simulink model "SingleStreamSSRwithPL"  (R2024a)
settings: Solver=VariableStepAuto  StartTime=0.0  StopTime=pow2(12)  RelTol=1e-3
PreLoadFcn:
  | xmcCheckSlxPath(bdroot);
  | SSR4withPL_init;
InitFcn:
  | xmcCheckSlxPath(bdroot);
  | SSR4withPL_init;
values from neighbouring files (symbols this model uses):
  SHIFT_ACC = 15    [SSR4withPL_init.m]
  T = N    (= 8)    [SSR4withPL_init.m]
  Taps = NormalizeCoef(UTaps,32768)    [SSR4withPL_init.m]
  VectorSize = FramesPerVector*N    (= 32)    [SSR4withPL_init.m]
undefined symbols (not defined in the file or in its folder): c, FIR_MultiKernel_cin, FIR_MultiKernel_cincout, FIR_MultiKernel_cout, S, SingleStream, vsva2197, xcvc1902
libraries: aieBasic x40, hdlBasic x40, aieUtilities x32, hdlUtilities x24, dspobslib x1, simulink x1, vmcUtilities x1
(part 1 of 3)
settings Model: Creator=oliviert  LastModifiedBy=robg
settings SolverCC: AlgebraicLoopSolver=TrustRegion
settings DebuggingCC: AlgebraicLoopMsg=none  UnconnectedInputMsg=warning  UnconnectedOutputMsg=warning  UnconnectedLineMsg=warning
settings ModelReferenceCC: EnableRefExpFcnMdlSchedulingChecks=on
settings RTWCC: GPUComputeCapability=3.5  DLArmComputeVersion=19.05

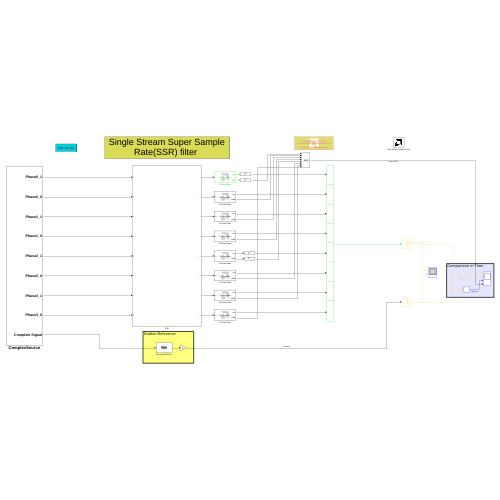
[thumbnail: Simulink's stored preview of the top-level diagram]
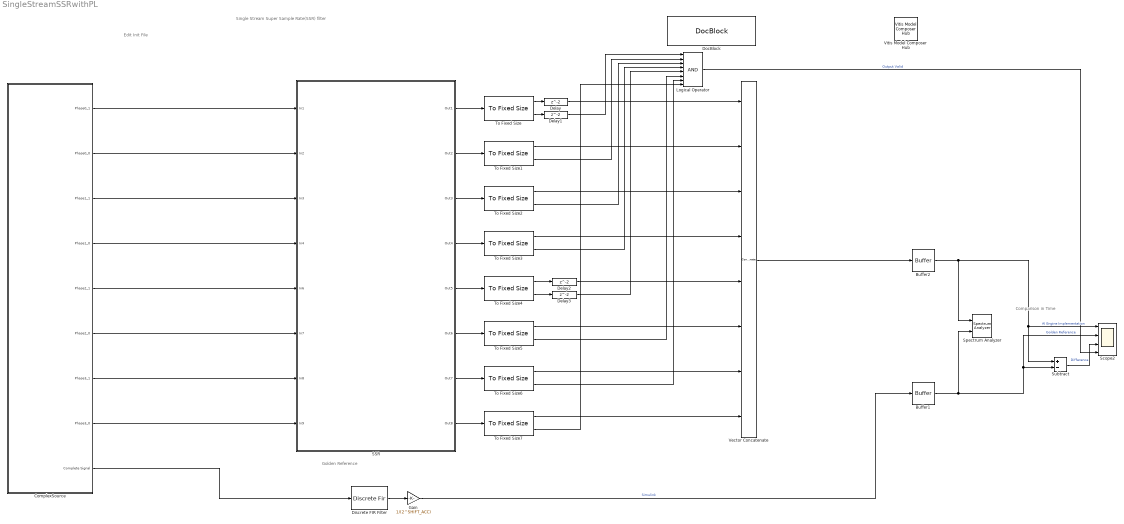
== system SingleStreamSSRwithPL ==
  note: Edit Init File
  note: Golden Reference
  note: Single Stream Super Sample Rate(SSR) filter
  note: Comparison in Time
  Buffer1 : Buffer  N=16  OutputFrames=off
  Buffer2 : Buffer  N=16  OutputFrames=off
  ComplexSource : Subsystem  mask{s=0}
      mask prompts: s "Seed"
  Delay{,1..3} (4 alike) : Delay
  Discrete FIR Filter : DiscreteFir  Coefficients=Taps  InputProcessing=Columns as channels (frame based)
  DocBlock : simulink/Model-Wide Utilities/DocBlock  DocumentType=Text  mask(DocBlock){}
      content=|
      | ///////////////////////////////////////////////////////////////////////////
      | // Copyright 2020 Xilinx
      | //
      | // Licensed under the Apache License, Version 2.0 (the "License");
      | // you may not use this file except in compliance with the License.
      | // You may obtain a copy of the License at
      | //
      | // http://www.apache.org/licenses/LICENSE-2.0
      | //
      | // Unless required by applicable law or agreed to in writing, software
      | // distributed under the License is distributed on an "AS IS" BASIS,
      | // WITHOUT WARRANTIES OR CONDITIONS OF ANY KIND, either express or implied.
      | // See the License for the specific language governing permissions and
      | // limitations under the License.
      | ///////////////////////////////////////////////////////////////////////////
      mask Display:
      | xmcDrawBlockIcon();
      | disp(['{\fontsize{10pt}(c) Copyright 2020' ' Xilinx, Inc.}\newline \newline '],'texmode','on');
      | disp('{\fontsize{10pt}Licensed under the Apache License 2.0}','texmode','on');
      | disp('\newline \newline \newline{\fontsize{10pt}Double Click for Copyright Notice}','texmode','on');
  Gain : Gain  Gain=1/(2^SHIFT_ACC)
  Logical Operator : Logic  Inputs=8  AllPortsSameDT=off  OutDataTypeStr=boolean
  SSR : Subsystem
  Scope2 : Scope  NumInputPorts=4
  Spectrum Analyzer : SpectrumAnalyzer  NumInputPorts=2  WindowPosition=[408.000000,320.000000,1093.000000,653.000000,]  Visible=on  ScopeFrameLocation=window  Method=Welch  SampleRate=8  Span=8  StartFrequency=-4  StopFrequency=4  AveragingMethod=Exponential  YLimits=[-15.9169 98.5393]  ShowLegend=on  ChannelNames="[\"\"]"  SelectedToolstripTab=spectrumAnalyzerToolstrip.spectrumTab  AllowFFTLengthLessThanSamplesPerUpdate=on  DefaultConfigurationName=spbscopes.SpectrumAnalyzerBlockCfg
  Subtract : Sum  Inputs=+-
  To Fixed Size{,1..7} (8 alike) : aieUtilities/To Fixed Size  Mode=Produce a valid output signal  OutputSize=Inherit: Same as input  CopyMethod=Buffer samples to form output  HasStatusOutput=on
  Vector Concatenate : Concatenate  NumInputs=8
  Vitis Model Composer Hub : vmcUtilities/Vitis Model Composer Hub  Tag=genX  CodeGeneration=off  SubsystemName=SSR  BlockHierPath=SingleStreamSSRwithPL/SSR  CompilationType=HWCompilation  SubsystemType=DUTNode  ExportTypeV2=HDL Netlist  AIEArrayConfig=Use entire AIE array  StartColumn=1  NumberOfColumns=1  TargetDirectory=./code  exportDesign=off  analyzeDesign=off  validateDesignOnHw=on  ExportType=HW Code  IpVendor=xilinx.com  IpLibrary=hls  IpVersion=1.0  IpHWLanguage=Verilog  AieCompilerOptions={}  AieSimulatorOptions={}  CreateTestbench=off  TestbenchStackSize=10  RunRtlSim=off  RunCSim=off  RunAieSim=on  AieSimTimeout=50000  RunAieSimProfiling=off  LaunchVitisAnalyzer=off  PlotOutput=off  RunX86Sim=off  X86SimTimeout=10  GenHwImage=off  GenLibadfXo=off  GenHwValidationCode=on  PlatformType=Not Specified  HwSystemType=Baremetal  HwValidationTarget=hw  ProjDevice=xcvc1902-vsva2197-1LP-e-S  ProjDevicePart=xcvc1902-vsva2197-1LP-e-S  AIEType=AIE  SamplePeriod=-1  ClockFrequency=200  DataPathParallelism=1  xilinxfamily=versalaicore  part=xcvc1902  speed=-1LP-e-S  package=vsva2197  directory=./code/ip/HDL_out/src  testbench=on  incr_netlist=off  synthesis_tool=Vivado  clock_wrapper=Clock Enables  dbl_ovrd=According to Block Masks  dcm_input_clock_period=10  sysclk_period=1e9/(570e6)  simulink_period=1  eval_field=0  IPInfoJsonString="{\"DUTSubsystemName\":\"SSR\",\"HDLSubsystem\":[{\"SubsystemName\":\"HDL_in\",\"IPName\":\"HDL_in\",\"IPLibrary\":\"VMC\",\"IPVendor\":\"User Company\",\"IPVersion\":\"1.0\",\"TargetDirectory\":\"./code\",\"SubsystemDir\":\"./code/ip/HDL_in\",\"FreqHz\":\"570000000\"},{\"SubsystemName\":\"HDL_out\",\"IPName\":\"HDL_out\",\"IPLibrary\":\"VMC\",\"IPVendor\":\"User Company\",\"IPVersion\":\"1.0\",\"TargetDirectory\":\"./code\",\"SubsystemDir\":\"./code/ip/HDL_out\",\"FreqHz\":\"570000000\"}],\"SubsystemTag\":\"DUTNode\",\"AIESubsystem\":{\"SubsystemName\":\"AI_Engine\",\"TargetDirectory\":\"./code\",\"AIEArrayConfig\":\"Use entire AIE array\",\"StartColumn\":\"0\",\"NumberOfColumns\":\"1\"}}"  LogFileName=/group/xcoswmktg2/robg/git/vfs/examples/hil/SingleStreamSSR_FIR_withHDL/code/model_composer.log  NThreads=4  IPConfigFile=/tmp/vmctmp-15379227158239209825/SingleStreamSSRwithPL_ipconfig.json
  wires:
  ComplexSource/9(Complete Signal) -> Discrete FIR Filter/1
  Discrete FIR Filter/1 -> Gain/1
  Subtract/1 -> Scope2/3  "Difference"
  Gain/1 -> Buffer1/1  "Simulink"
  Buffer1/1 -> Subtract/2, Scope2/2, Spectrum Analyzer/2  "Golden Reference"
  Buffer2/1 -> Subtract/1, Scope2/1, Spectrum Analyzer/1  "AI Engine Implementation"
  ComplexSource/1(Phase0_1) -> SSR/1(In1)
  ComplexSource/2(Phase0_0) -> SSR/2(In2)
  ComplexSource/3(Phase1_1) -> SSR/3(In3)
  ComplexSource/4(Phase1_0) -> SSR/4(In4)
  ComplexSource/5(Phase2_1) -> SSR/5(In6)
  ComplexSource/6(Phase2_0) -> SSR/6(In7)
  ComplexSource/7(Phase3_1) -> SSR/7(In8)
  ComplexSource/8(Phase3_0) -> SSR/8(In9)
  SSR/1(Out1) -> To Fixed Size/1
  SSR/2(Out2) -> To Fixed Size1/1
  SSR/3(Out3) -> To Fixed Size2/1
  SSR/4(Out4) -> To Fixed Size3/1
  SSR/5(Out5) -> To Fixed Size4/1
  SSR/6(Out6) -> To Fixed Size5/1
  SSR/7(Out7) -> To Fixed Size6/1
  SSR/8(Out8) -> To Fixed Size7/1
  To Fixed Size/2 -> Delay1/1
  To Fixed Size1/2 -> Logical Operator/2
  To Fixed Size2/2 -> Logical Operator/3
  To Fixed Size3/2 -> Logical Operator/4
  To Fixed Size4/2 -> Delay3/1
  To Fixed Size5/2 -> Logical Operator/6
  To Fixed Size6/2 -> Logical Operator/7
  To Fixed Size7/2 -> Logical Operator/8
  To Fixed Size/1 -> Delay/1
  To Fixed Size5/1 -> Vector Concatenate/6
  To Fixed Size4/1 -> Delay2/1
  To Fixed Size1/1 -> Vector Concatenate/2
  To Fixed Size2/1 -> Vector Concatenate/3
  Vector Concatenate/1 -> Buffer2/1
  To Fixed Size7/1 -> Vector Concatenate/8
  To Fixed Size3/1 -> Vector Concatenate/4
  To Fixed Size6/1 -> Vector Concatenate/7
  Logical Operator/1 -> Scope2/4  "Output Valid"
  Delay/1 -> Vector Concatenate/1
  Delay1/1 -> Logical Operator/1
  Delay3/1 -> Logical Operator/5
  Delay2/1 -> Vector Concatenate/5

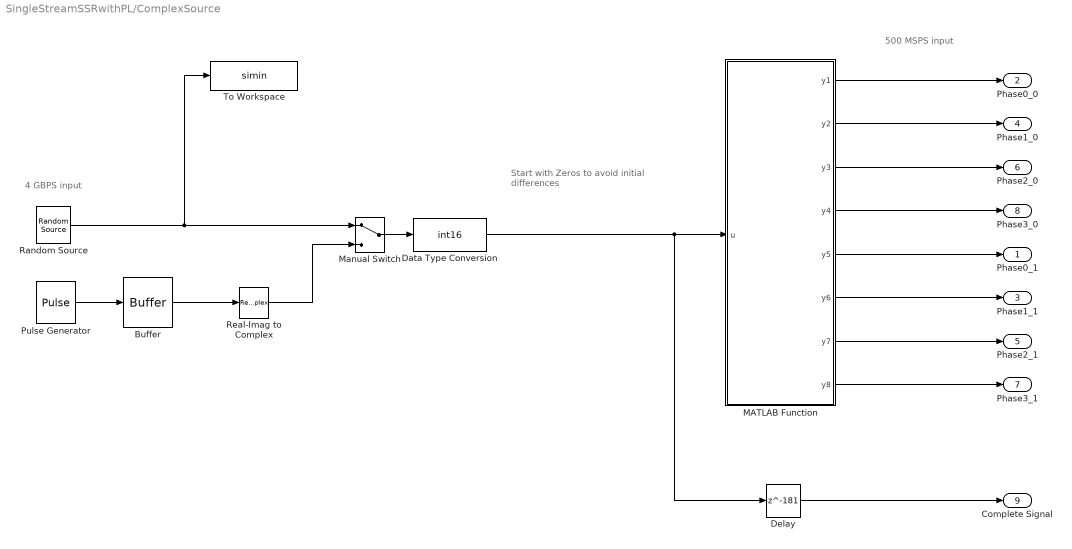
== system SingleStreamSSRwithPL/ComplexSource ==
  note: Start with Zeros
      | to avoid
      | initial differences
  note: 4 GBPS input
  note: 500 MSPS input
  Buffer : Buffer  N=VectorSize  OutputFrames=off
  Data Type Conversion : DataTypeConversion  OutDataTypeStr=int16  SaturateOnIntegerOverflow=off  RndMeth=Floor
  Delay : Delay  DelayLength=181  InputProcessing=Columns as channels (frame based)
  MATLAB Function : MATLAB Function  TreatAsAtomicUnit=on
  Manual Switch : ManualSwitch
  Pulse Generator : DiscretePulseGenerator  Amplitude=20000  Period=32 + 40*5  PhaseDelay=32  SampleTime=1/T
  Random Source : dspobslib/Random Source  SrcType=Uniform  NormMethod=Ziggurat  CltLength=12  MinVal=-20000  MaxVal=20000  MeanVal=0  VarVal=1  RepMode=Specify seed  rawSeed=s  IsInherit=off  SampMode=Discrete  SampTime=1/T  SampFrame=VectorSize  DataType=Double  OutComplex=Complex  OutputFrames=off
  Real-Imag to Complex : RealImagToComplex  Input=Real
  To Workspace : ToWorkspace  VariableName=simin  SaveFormat=Timeseries  SampleTime=-1
  Phase0_1 : Outport
  Phase0_0 : Outport  Port=2
  Phase1_1 : Outport  Port=3
  Phase1_0 : Outport  Port=4
  Phase2_1 : Outport  Port=5
  Phase2_0 : Outport  Port=6
  Phase3_1 : Outport  Port=7
  Phase3_0 : Outport  Port=8
  Complete Signal : Outport  Port=9
  wires:
  MATLAB Function/1(y1) -> Phase0_0/1
  MATLAB Function/2(y2) -> Phase1_0/1
  MATLAB Function/3(y3) -> Phase2_0/1
  MATLAB Function/4(y4) -> Phase3_0/1
  Real-Imag to Complex/1 -> Manual Switch/2
  Pulse Generator/1 -> Buffer/1
  Delay/1 -> Complete Signal/1
  Buffer/1 -> Real-Imag to Complex/1
  Manual Switch/1 -> Data Type Conversion/1
  MATLAB Function/8(y8) -> Phase3_1/1
  MATLAB Function/7(y7) -> Phase2_1/1
  MATLAB Function/6(y6) -> Phase1_1/1
  MATLAB Function/5(y5) -> Phase0_1/1
  Random Source/1 -> To Workspace/1, Manual Switch/1
  Data Type Conversion/1 -> Delay/1, MATLAB Function/1(u)

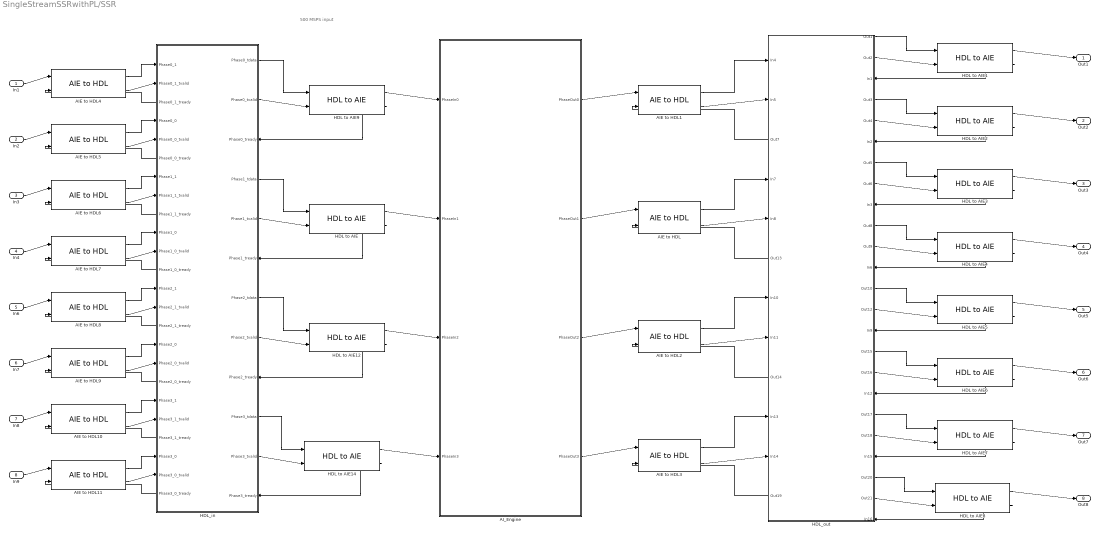
== system SingleStreamSSRwithPL/SSR ==
  note: 500 MSPS input
  In1 : Inport
  In2 : Inport  Port=2
  In3 : Inport  Port=3
  In4 : Inport  Port=4
  In6 : Inport  Port=5
  In7 : Inport  Port=6
  In8 : Inport  Port=7
  In9 : Inport  Port=8
  AIE to HDL{,1..3} (4 alike) : aieUtilities/AIE to HDL  OutDataType=uint64  OutSampleTime=1
  AIE to HDL{4..11} (8 alike) : aieUtilities/AIE to HDL  OutDataType=uint32  OutSampleTime=Inherit: Same as tready
  AI_Engine : Subsystem
  HDL to AIE{,9,12,14} (4 alike) : aieUtilities/HDL to AIE  InDataType=uint32  OutDataType=int16 (c)  OutSampleTime=4/T  SamplesPerFrame=4  RateReduceFactor=1  ManuallySpecifyOutSampleTime=on
  HDL to AIE{1..8} (8 alike) : aieUtilities/HDL to AIE  InDataType=uint32  OutDataType=int16 (c)  OutSampleTime=1  SamplesPerFrame=1  RateReduceFactor=1  ManuallySpecifyOutSampleTime=on
  HDL_in : Subsystem
      settings: PortSchema="{\"entries\":[{\"content\":{\"sides\":[{\"content\":{\"connectorIds\":[\"In1\",\"In2\",\"Out9\",\"In3\",\"In4\",\"Out10\",\"In5\",\"In6\",\"Out11\",\"In7\",\"In8\",\"Out12\",\"In9\",\"In10\",\"Out13\",\"In11\",\"In12\",\"Out14\",\"In13\",\"In14\",\"Out15\",\"In15\",\"In16\",\"Out16\"]},\"type\":\"ConnectorPlacement.EquallySpacedRectSide\",\"uuid\":\"43963710-6fd6-4ca2-aef5-f578b9dcb653\"},{\"content\":{\"connectorIds\":[\"Out1\",\"Out2\",\"In17\",\"Out3\",\"Out4\",\"In18\",\"Out5\",\"Out6\",\"In19\",\"Out7\",\"Out8\",\"In20\"],\"side\":\"RIGHT\"},\"type\":\"ConnectorPlacement.EquallySpacedRectSide\",\"uuid\":\"a4fb1d0d-700c-40f1-8501-f280c21d0c52\"},{\"content\":{\"connectorIds\":[],\"side\":\"TOP\"},\"type\":\"ConnectorPlacement.EquallySpacedRectSide\",\"uuid\":\"ff581830-d8dd-44d7-ae40-7c0c1ac080ec\"}]},\"type\":\"ConnectorPlacement.EquallySpacedConnector\",\"uuid\":\"e2183898-06e4-482e-ae06-3d392b216275\"}],\"packageUris\":[\"http://schema.mathworks.com/mf0/Connector/R2020b\"],\"version\":\"1.0\"}"
  HDL_out : Subsystem
      settings: PortSchema="{\"entries\":[{\"content\":{\"sides\":[{\"content\":{\"connectorIds\":[\"In1\",\"In2\",\"Out17\",\"In3\",\"In4\",\"Out18\",\"In5\",\"In6\",\"Out19\",\"In7\",\"In8\",\"Out20\"]},\"type\":\"ConnectorPlacement.EquallySpacedRectSide\",\"uuid\":\"cedaa4bc-2afe-4f55-8e95-e7c88c9ac45d\"},{\"content\":{\"connectorIds\":[\"Out1\",\"Out2\",\"In9\",\"Out3\",\"Out4\",\"In10\",\"Out5\",\"Out6\",\"In11\",\"Out7\",\"Out8\",\"In12\",\"Out9\",\"Out10\",\"In13\",\"Out11\",\"Out12\",\"In14\",\"Out13\",\"Out14\",\"In15\",\"Out15\",\"Out16\",\"In16\"],\"side\":\"RIGHT\"},\"type\":\"ConnectorPlacement.EquallySpacedRectSide\",\"uuid\":\"25527022-5cc7-4db8-977d-2f658874d9e0\"},{\"content\":{\"connectorIds\":[],\"side\":\"TOP\"},\"type\":\"ConnectorPlacement.EquallySpacedRectSide\",\"uuid\":\"b8c7a8f8-1c08-473a-8336-759f79ea6c23\"}]},\"type\":\"ConnectorPlacement.EquallySpacedConnector\",\"uuid\":\"354f3813-e5f3-40c4-8c5f-540088327230\"}],\"packageUris\":[\"http://schema.mathworks.com/mf0/Connector/R2020b\"],\"version\":\"1.0\"}"
  Out1 : Outport
  Out2 : Outport  Port=2
  Out3 : Outport  Port=3
  Out4 : Outport  Port=4
  Out5 : Outport  Port=5
  Out6 : Outport  Port=6
  Out7 : Outport  Port=7
  Out8 : Outport  Port=8
  wires:
  AIE to HDL5/1 -> HDL_in/3(Phase0_0)
  HDL to AIE/1 -> AI_Engine/2(PhaseIn1)
  HDL to AIE12/1 -> AI_Engine/3(PhaseIn2)
  AI_Engine/1(PhaseOut0) -> AIE to HDL1/1
  HDL to AIE14/1 -> AI_Engine/4(PhaseIn3)
  AI_Engine/3(PhaseOut2) -> AIE to HDL2/1
  AIE to HDL5/2 -> HDL_in/4(Phase0_0_tvalid)
  HDL_in/10(Phase0_0_tready) -> AIE to HDL5/2
  In2/1 -> AIE to HDL5/1
  In3/1 -> AIE to HDL6/1
  AIE to HDL6/1 -> HDL_in/5(Phase1_1)
  AIE to HDL6/2 -> HDL_in/6(Phase1_1_tvalid)
  HDL_in/11(Phase1_1_tready) -> AIE to HDL6/2
  In4/1 -> AIE to HDL7/1
  AIE to HDL7/1 -> HDL_in/7(Phase1_0)
  AIE to HDL7/2 -> HDL_in/8(Phase1_0_tvalid)
  HDL_in/12(Phase1_0_tready) -> AIE to HDL7/2
  In6/1 -> AIE to HDL8/1
  AIE to HDL8/1 -> HDL_in/9(Phase2_1)
  AIE to HDL8/2 -> HDL_in/10(Phase2_1_tvalid)
  HDL_in/13(Phase2_1_tready) -> AIE to HDL8/2
  In7/1 -> AIE to HDL9/1
  AIE to HDL9/1 -> HDL_in/11(Phase2_0)
  AIE to HDL9/2 -> HDL_in/12(Phase2_0_tvalid)
  HDL_in/14(Phase2_0_tready) -> AIE to HDL9/2
  In8/1 -> AIE to HDL10/1
  AIE to HDL10/1 -> HDL_in/13(Phase3_1)
  AIE to HDL10/2 -> HDL_in/14(Phase3_1_tvalid)
  HDL_in/15(Phase3_1_tready) -> AIE to HDL10/2
  In9/1 -> AIE to HDL11/1
  AIE to HDL11/1 -> HDL_in/15(Phase3_0)
  AIE to HDL11/2 -> HDL_in/16(Phase3_0_tvalid)
  HDL_in/16(Phase3_0_tready) -> AIE to HDL11/2
  HDL_in/9(Phase0_1_tready) -> AIE to HDL4/2
  AIE to HDL4/1 -> HDL_in/1(Phase0_1)
  AIE to HDL4/2 -> HDL_in/2(Phase0_1_tvalid)
  In1/1 -> AIE to HDL4/1
  AI_Engine/4(PhaseOut3) -> AIE to HDL3/1
  HDL to AIE1/1 -> Out1/1
  HDL to AIE2/1 -> Out2/1
  HDL to AIE3/1 -> Out3/1
  HDL to AIE4/1 -> Out4/1
  HDL to AIE5/1 -> Out5/1
  HDL to AIE7/1 -> Out7/1
  HDL to AIE8/1 -> Out8/1
  HDL to AIE1/2 -> HDL_out/9(In1)
  HDL to AIE2/2 -> HDL_out/10(In2)
  HDL to AIE3/2 -> HDL_out/11(In3)
  AIE to HDL1/1 -> HDL_out/1(In4)
  AIE to HDL1/2 -> HDL_out/2(In5)
  HDL to AIE4/2 -> HDL_out/12(In6)
  AIE to HDL/1 -> HDL_out/3(In7)
  AIE to HDL/2 -> HDL_out/4(In8)
  HDL to AIE5/2 -> HDL_out/13(In9)
  AIE to HDL2/1 -> HDL_out/5(In10)
  AIE to HDL2/2 -> HDL_out/6(In11)
  HDL to AIE6/2 -> HDL_out/14(In12)
  AIE to HDL3/1 -> HDL_out/7(In13)
  AIE to HDL3/2 -> HDL_out/8(In14)
  HDL to AIE7/2 -> HDL_out/15(In15)
  HDL to AIE8/2 -> HDL_out/16(In16)
  HDL_out/1(Out1) -> HDL to AIE1/1
  HDL_out/2(Out2) -> HDL to AIE1/2
  HDL_out/3(Out3) -> HDL to AIE2/1
  HDL_out/4(Out4) -> HDL to AIE2/2
  HDL_out/5(Out5) -> HDL to AIE3/1
  HDL_out/6(Out6) -> HDL to AIE3/2
  HDL_out/17(Out7) -> AIE to HDL1/2
  HDL_out/7(Out8) -> HDL to AIE4/1
  HDL_out/8(Out9) -> HDL to AIE4/2
  HDL_out/9(Out10) -> HDL to AIE5/1
  HDL_out/10(Out12) -> HDL to AIE5/2
  HDL_out/18(Out13) -> AIE to HDL/2
  HDL_out/19(Out14) -> AIE to HDL2/2
  HDL_out/11(Out15) -> HDL to AIE6/1
  HDL_out/12(Out16) -> HDL to AIE6/2
  HDL_out/13(Out17) -> HDL to AIE7/1
  HDL_out/14(Out18) -> HDL to AIE7/2
  HDL_out/20(Out19) -> AIE to HDL3/2
  HDL_out/15(Out20) -> HDL to AIE8/1
  HDL_out/16(Out21) -> HDL to AIE8/2
  AI_Engine/2(PhaseOut1) -> AIE to HDL/1
  HDL_in/3(Phase1_tdata) -> HDL to AIE/1
  HDL_in/4(Phase1_tvalid) -> HDL to AIE/2
  HDL_in/5(Phase2_tdata) -> HDL to AIE12/1
  HDL_in/6(Phase2_tvalid) -> HDL to AIE12/2
  HDL_in/7(Phase3_tdata) -> HDL to AIE14/1
  HDL_in/8(Phase3_tvalid) -> HDL to AIE14/2
  HDL to AIE9/1 -> AI_Engine/1(PhaseIn0)
  HDL to AIE12/2 -> HDL_in/19(Phase2_tready)
  HDL to AIE14/2 -> HDL_in/20(Phase3_tready)
  HDL_in/1(Phase0_tdata) -> HDL to AIE9/1
  HDL to AIE/2 -> HDL_in/18(Phase1_tready)
  HDL_in/2(Phase0_tvalid) -> HDL to AIE9/2
  HDL to AIE9/2 -> HDL_in/17(Phase0_tready)
  HDL to AIE6/1 -> Out6/1
